simulink model "Actuator_FO_TestBed_org"  (Simulink 10.0)
settings: Solver=ode4  StartTime=0.0  StopTime=10  FixedStep=0.2  RelTol=1e-3  EnableMultiTasking=on
undefined symbols (not defined in the file): MWS
libraries: Lib_Cntrl_FirstOrderActuator_TMATS x1
settings Model: Creator=jwchapm2  LastModifiedBy=annonymous
settings DataIOCC: LimitDataPoints=on
settings OptimizationCC: ExpressionDepthLimit=2147483647
settings DebuggingCC: SolverPrmCheckMsg=warning  StateNameClashWarn=warning
settings GRTTargetCC: GeneratePreprocessorConditionals=Disable all  CombineOutputUpdateFcns=on  GRTInterface=off
settings ConfigComp: CovExternalEMLEnable=off

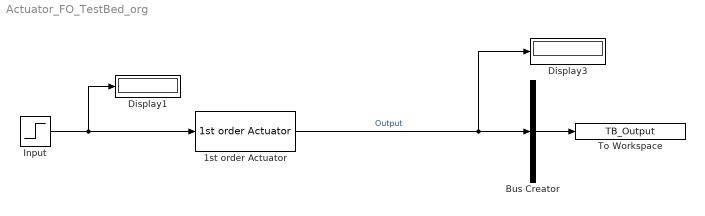
== system Actuator_FO_TestBed_org ==
  1st order Actuator : Lib_Cntrl_FirstOrderActuator_TMATS/1st order Actuator  Gain_M=MWS.Actuator_FO.Gain  Tau_M=MWS.Actuator_FO.Tau  IC_M=0  MaxSat_M=MWS.Actuator_FO.max  MinSat_M=MWS.Actuator_FO.min  deadband_M=MWS.Actuator_FO.DeadBand  rateLimit_M=MWS.Actuator_FO.RateLim
  Bus Creator : BusCreator  Inputs=1
  Display1 : Display
  Display3 : Display
  Input : Step  Time=MWS.Actuator_FO.Step_Time  Before=MWS.Actuator_FO.Step_IV  After=MWS.Actuator_FO.Inp  SampleTime=0
  To Workspace : ToWorkspace  VariableName=TB_Output  SampleTime=-1
  wires:
  1st order Actuator/1 -> Display3/1, Bus Creator/1  "Output"
  Bus Creator/1 -> To Workspace/1
  Input/1 -> 1st order Actuator/1, Display1/1
